simulink model "autoMBD_example_PI_ObjectiveDD"  (R2020b)
settings: Solver=FixedStepAuto  StartTime=0.0  StopTime=10.0  FixedStep=0.001  RelTol=1e-3
values from neighbouring files (symbols this model uses):
  Param_Ki = 3.0    [PI_ObjectiveDD.sldd]
  Param_Kp = 1.0    [PI_ObjectiveDD.sldd]
undefined symbols (not defined in the file or in its folder): DiscIntNeverNeededParam
settings Model: DataDictionary=PI_ObjectiveDD.sldd  EnableAccessToBaseWorkspace=off  Creator=k  LastModifiedBy=k
settings OptimizationCC: DefaultParameterBehavior=Inlined  EnhancedBackFolding=on  PassReuseOutputArgsAs=Individual arguments  ZeroExternalMemoryAtStartup=off  ZeroInternalMemoryAtStartup=off  OptimizeBlockOrder=speed  DifferentSizesBufferReuse=on  OptimizationCustomize=off  EfficientTunableParamExpr=on
settings DebuggingCC: ParameterTunabilityLossMsg=error
settings SFSimCC: MATLABDynamicMemAlloc=off
settings RTWCC: Description=Embedded Coder  SystemTargetFile=ert.tlc  GenCodeOnly=on  TemplateMakefile=ert_default_tmf
settings CodeAppCC: ForceParamTrailComments=on  IgnoreCustomStorageClasses=off  MaxIdLength=63  OperatorAnnotations=on  SimulinkDataObjDesc=on  SFDataObjDesc=on  InsertBlockDesc=on
settings ERTTargetCC: TargetLangStandard=C99 (ISO)  GenerateSampleERTMain=on  InlinedParameterPlacement=NonHierarchical  ERTCustomFileTemplate=example_file_process.tlc  MaxLineWidth=300

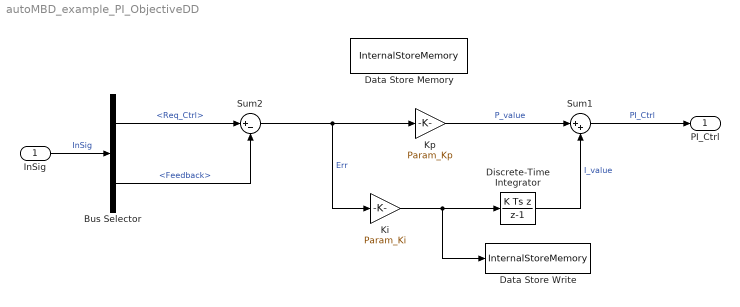
== system autoMBD_example_PI_ObjectiveDD ==
  InSig : Inport  OutDataTypeStr=Bus: InputBus
  Bus Selector : BusSelector  OutputSignals=Req_Ctrl,Feedback
  Data Store Memory : DataStoreMemory  DataStoreName=InternalStoreMemory  ReadBeforeWriteMsg=warning  WriteAfterWriteMsg=warning  WriteAfterReadMsg=warning  ShowAdditionalParam=off  StateMustResolveToSignalObject=on
  Data Store Write : DataStoreWrite  DataStoreName=InternalStoreMemory
  Discrete-Time Integrator : DiscreteIntegrator  IntegratorMethod=Integration: Backward Euler  SampleTime=-1  StateName=DiscIntegState  ICPrevOutput=DiscIntNeverNeededParam  ICPrevScaledInput=DiscIntNeverNeededParam  StateMustResolveToSignalObject=on
  Ki : Gain  Gain=Param_Ki
  Kp : Gain  Gain=Param_Kp
  Sum1 : Sum  Inputs=|++
  Sum2 : Sum  Inputs=|+-
  PI_Ctrl : Outport  SignalName=OutSig
      settings: MustResolveToSignalObject=on
  wires:
  Sum1/1 -> PI_Ctrl/1  "PI_Ctrl"
  Bus Selector/2 -> Sum2/2  "<Feedback>"
  Bus Selector/1 -> Sum2/1  "<Req_Ctrl>"
  Sum2/1 -> Ki/1, Kp/1  "Err"
  Kp/1 -> Sum1/1  "P_value"
  Ki/1 -> Data Store Write/1, Discrete-Time Integrator/1
  Discrete-Time Integrator/1 -> Sum1/2  "I_value"
  InSig/1 -> Bus Selector/1  "InSig"
